simulink model "Mod5_model"  (R2020a)
settings: Solver=VariableStepAuto  StartTime=0.0  StopTime=10.0  RelTol=1e-3
settings Model: DataDictionary=clutch_datadict.sldd  Creator=kiran  LastModifiedBy=kiran

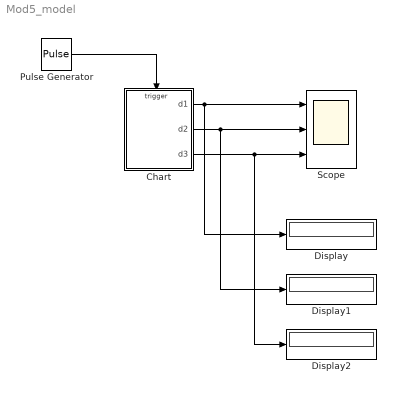
== system Mod5_model ==
  Chart : Stateflow chart  TreatAsAtomicUnit=on
  Display : Display
  Display1 : Display
  Display2 : Display
  Pulse Generator : DiscretePulseGenerator  PulseType=Time based  Period=0.1  PulseWidth=5
  Scope : Scope  NumInputPorts=3
  wires:
  Pulse Generator/1 -> Chart/Trigger
  Chart/1(d1) -> Display/1, Scope/1
  Chart/2(d2) -> Display1/1, Scope/2
  Chart/3(d3) -> Display2/1, Scope/3

== stateflow chart Mod5_model/Chart ==
  state digit1 [parallel]
    settings: executionOrder=1
    state One
      en:d1=1;
    state zero
      en:d1=0;
    state Two
      en:d1=2;
    state Four
      en:d1=4;
    state Three
      en:d1=3;
    digit1.zero -> digit1.One : ic1
    digit1.One -> digit1.Two : ic1
    (default) -> digit1.zero
    digit1.Four -> digit1.zero : ic1/{ic2}
    digit1.Two -> digit1.Three : ic1
    digit1.Three -> digit1.Four : ic1
  state digit2 [parallel]
    settings: executionOrder=2
    state One
      en:d2=1;
    state zero
      en:d2=0;
    state Two
      en:d2=2;
    state Four
      en:d2=4;
    state Three
      en:d2=3;
    digit2.zero -> digit2.One : ic2
    digit2.One -> digit2.Two : ic2
    (default) -> digit2.zero
    digit2.Four -> digit2.zero : ic2/{ic3}
    digit2.Two -> digit2.Three : ic2
    digit2.Three -> digit2.Four : ic2
  state digit3 [parallel]
    settings: executionOrder=3
    state One
      en:d3=1;
    state zero
      en:d3=0;
    state Two
      en:d3=2;
    state Four
      en:d3=4;
    state Three
      en:d3=3;
    digit3.zero -> digit3.One : ic3
    digit3.One -> digit3.Two : ic3
    (default) -> digit3.zero
    digit3.Four -> digit3.zero : ic3
    digit3.Two -> digit3.Three : ic3
    digit3.Three -> digit3.Four : ic3
  data: d1 output; d2 output; d3 output
  events: ic2 local FUNCTION_CALL_EVENT; ic3 local FUNCTION_CALL_EVENT; ic1 input RISING_EDGE_EVENT
